simulink model "IRB140"  (R2016b)
settings: Solver=ode113  StartTime=0.0  StopTime=40  RelTol=1e-3
(part 9 of 9)

== matlab function IRB140/outer loop1 ==
  data: e_theta input; e_thetad input; thetadd_desired input; aq output; nW output
function [aq, nW] = fcn(e_theta, e_thetad,thetadd_desired)
e = [e_theta; e_thetad];
wn = 10;
Kp = diag(ones(6,1)*wn^2);
Kd = diag(ones(6,1)*2*wn);
Ro = 10*(norm(e) + norm(e)^2 + 1);

A = [zeros(6) eye(6); -Kp -Kd];
B = [zeros(6); eye(6)];

% Q = eye(12);
% P = lyap(A,Q);
P = [1.5000 0 0 0 0 0 -0.5000 0 0 0 0 0; 0 1.5000 0 0 0 0 0 -0.5000 0 0 0 0; 0 0 1.5000 0 0 0 0 0 -0.5000 0 0 0; ...
     0 0 0 1.5000 0 0 0 0 0 -0.5000 0 0; 0 0 0 0 1.5000 0 0 0 0 0 -0.5000 0; 0 0 0 0 0 1.5000 0 0 0 0 0 -0.5000; ...
     -0.5000 0 0 0 0 0 0.5000 0 0 0 0 0; 0 -0.5000 0 0 0 0 0 0.5000 0 0 0 0; 0 0 -0.5000 0 0 0 0 0 0.5000 0 0 0; ...
     0 0 0 -0.5000 0 0 0 0 0 0.5000 0 0; 0 0 0 0 -0.5000 0 0 0 0 0 0.5000 0; 0 0 0 0 0 -0.5000 0 0 0 0 0 0.5000];
W = transpose(B)*P*e;
eps = 0;
if norm(W) > eps
    delta = -Ro*W/norm(W);
else
    if eps == 0
        delta = 0;
    else
        delta = -Ro*W/eps;
    end
end

aq = thetadd_desired - Kd*e_thetad - Kp*e_theta + delta;
nW = norm(W);
